simulink subsystem "ball_out_of_bounds_detector"  (R2022b)
settings: Solver=VariableStepAuto  StartTime=0.0  StopTime=10.0  RelTol=1e-3
settings Model: Creator=User  LastModifiedBy=User

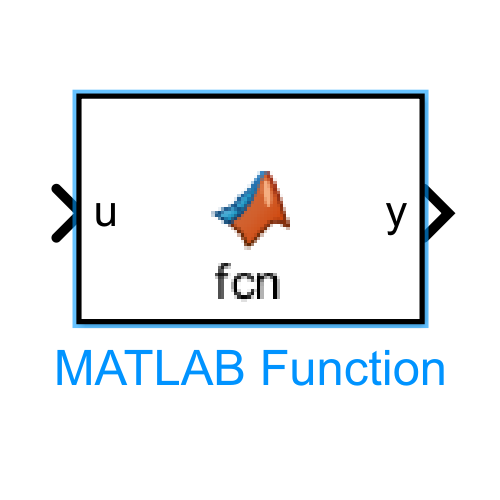
[thumbnail: Simulink's stored preview of the top-level diagram]
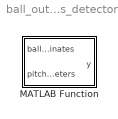
== system ball_out_of_bounds_detector ==
  MATLAB Function : MATLAB Function  TreatAsAtomicUnit=on

== matlab function ball_out_of_bounds_detector/MATLAB Function ==
  data: ball_coordinates input; y output; pitch_parameters input
function y = ballOutOfBoundsDetector(ball_coordinates, pitch_parameters)

% Set up field parameters
pitch_width = pitch_parameters(2);

y = 1; % 1 is normal game state

if (ball_coordinates(2) > pitch_width/2) || (ball_coordinates(2) < (-pitch_width/2))
    y = 5; % 5 is ball out of bounds state
end
